simulink model "ChiefMaster_TTC580"  (R2022b)
settings: Solver=FixedStepAuto  StartTime=0.0  StopTime=10  FixedStep=0.01  RelTol=1e-3
values from neighbouring files (symbols this model uses):
  BattBox1_No = single(1)    [Parameters.m]
  BattBox2_No = single(2)    [Parameters.m]
  BattBox3_No = single(3)    [Parameters.m]
  CurrentLB = single(-3)    [Parameters.m]
  CurrentReductionConstant_Lvl0 = single(0.03)    [Parameters.m]
  CurrentReductionConstant_Lvl1 = single(0.05)    [Parameters.m]
  CurrentReductionConstant_Lvl2 = single(0.07)    [Parameters.m]
  CurrentReductionConstant_Lvl3 = single(0.1)    [Parameters.m]
  CurrentUB = single(3)    [Parameters.m]
  DCHV_Minus_In_Delay_ms = single(500)    [Parameters.m]
  FL_sHVC_CellBalanceVoltage_mV = single(3500)    [Parameters.m]
  FL_sInrushCurrent_dividebyzero = single(0.00001)    [Parameters.m]
  FL_u8HMI_BuzzerTimer = uint8(3)    [Parameters.m]
  IP_boActValue = true    [Parameters.m]
  IP_boDeactValue = false    [Parameters.m]
  IP_boInitValue = false    [Parameters.m]
  IP_s_LB = 18000    [Parameters.m]
  IP_s_UB = 22000    [Parameters.m]
  IP_sBatt1_ChargeCurrentMax_Factor = single(0.1)    [Parameters.m]
  IP_sBatt1_ChargeCurrentMax_LB = single(0)    [Parameters.m]
  IP_sBatt1_ChargeCurrentMax_Offset = single(0)    [Parameters.m]
  IP_sBatt1_ChargeCurrentMax_UB = single(6553.5)    [Parameters.m]
  IP_sBatt1_Current_Factor = single(0.1)    [Parameters.m]
  IP_sBatt1_Current_LB = single(-3276.8)    [Parameters.m]
  IP_sBatt1_Current_Offset = single(0)    [Parameters.m]
  IP_sBatt1_Current_UB = single(3276.8)    [Parameters.m]
  IP_sBatt1_DisChargeCurrentMax_Factor = single(0.1)    [Parameters.m]
  IP_sBatt1_DisChargeCurrentMax_LB = single(0)    [Parameters.m]
  IP_sBatt1_DisChargeCurrentMax_Offset = single(0)    [Parameters.m]
  IP_sBatt1_DisChargeCurrentMax_UB = single(6553.5)    [Parameters.m]
  IP_sBatt1_InsulationResistance_Factor = single(5)    [Parameters.m]
  IP_sBatt1_InsulationResistance_LB = single(0)    [Parameters.m]
  IP_sBatt1_InsulationResistance_Offset = single(0)    [Parameters.m]
  IP_sBatt1_InsulationResistance_UB = single(0)    [Parameters.m]
  IP_sBatt1_LiBa_IntResist_mOhm = single(25)    [Parameters.m]
  IP_sBatt1_SOC_Factor = single(1)    [Parameters.m]
  IP_sBatt1_SOC_LB = single(0)    [Parameters.m]
  IP_sBatt1_SOC_Offset = single(0)    [Parameters.m]
  IP_sBatt1_SOC_UB = single(100)    [Parameters.m]
  IP_sBatt1_SOH_Factor = single(1)    [Parameters.m]
  IP_sBatt1_SOH_LB = single(0)    [Parameters.m]
  IP_sBatt1_SOH_Offset = single(0)    [Parameters.m]
  IP_sBatt1_SOH_UB = single(100)    [Parameters.m]
  IP_sBatt1_Ubatt_Factor = single(0.1)    [Parameters.m]
  IP_sBatt1_Ubatt_LB = single(0)    [Parameters.m]
  IP_sBatt1_Ubatt_Offset = single(0)    [Parameters.m]
  IP_sBatt1_Ubatt_UB = single(6553.5)    [Parameters.m]
  IP_sBatt1_UserRi_Factor = single(1)    [Parameters.m]
  IP_sBatt1_UserRi_LB = single(0)    [Parameters.m]
  IP_sBatt1_UserRi_Offset = single(0)    [Parameters.m]
  IP_sBatt1_UserRi_UB = single(255)    [Parameters.m]
  IP_sBatt1_VoltageAtSensor_Factor = single(0.02)    [Parameters.m]
  IP_sBatt1_VoltageAtSensor_LB = single(0)    [Parameters.m]
  IP_sBatt1_VoltageAtSensor_Offset = single(0)    [Parameters.m]
  IP_sBatt1_VoltageAtSensor_UB = single(1310.7)    [Parameters.m]
  IP_sBatt2_LiBa_IntResist_mOhm = single(25)    [Parameters.m]
  IP_sBatt3_LiBa_IntResist_mOhm = single(25)    [Parameters.m]
  IP_sEM_LB = 2000    [Parameters.m]
  IP_sEM_UB = 8000    [Parameters.m]
  IP_sFB_LB = 5000    [Parameters.m]
  IP_sFB_UB = 10000    [Parameters.m]
  IP_sHVIL_LB = 12000    [Parameters.m]
  IP_sHVIL_UB = 15000    [Parameters.m]
  IP_sLoad_Voltage_Factor = single(1)    [Parameters.m]
  IP_sLoad_Voltage_LB = single(0)    [Parameters.m]
  IP_sLoad_Voltage_Offset = single(0)    [Parameters.m]
  IP_sLoad_Voltage_UB = single(65535)    [Parameters.m]
  IP_u8HVIL_Delay_ms = uint8(100)    [Parameters.m]
  IP_u8HW_IN_delay_ms = uint8(100)    [Parameters.m]
  IT_sInsulationSafeValue_kOhm = single(650)    [Parameters.m]
  IT_u8IMD_DelayTime_s = uint8(20)    [Parameters.m]
  MainHV_Minus_In_Delay = single(5)    [Parameters.m]
  MainHV_StatusDelay = single(5)    [Parameters.m]
  NotAvailable_uint16 = single(65535)    [Parameters.m]
  NotAvailable_uint8 = uint8(255)    [Parameters.m]
  OP_boHVIL_Supply = boolean(1)    [Parameters.m]
  SafeCurrentToCloseHV_A = single(5)    [Parameters.m]
  SafeVoltageToCloseHV_V = single(0.5)    [Parameters.m]
  UnexpectedBattChargingFcn_Available = boolean(1)    [Parameters.m]
  Voltage_NA_UB = uint16(65535)    [Parameters.m]
  VoltageSensorAvailableBB1 = boolean(0)    [Parameters.m]
  VoltageSensorAvailableBB2 = boolean(0)    [Parameters.m]
  VoltageSensorAvailableBB3 = boolean(0)    [Parameters.m]
libraries: simulink x184, Library_DataProcessing_v1_1 x167, Library_DataProcessing_v1 x142, libCM x28
(part 18 of 19)

== system ChiefMaster_TTC580/ChiefMaster/Input Processing/LiBa/LiBa_Box3/BMS_InsulationMonitor/Subsystem ==
  byte0 : Inport
  byte1 : Inport  Port=2
  C_LB_BMS_InsulationMonitor_Timeout : Inport  Port=3
  Bus Creator : BusCreator  Inputs=3
  Constant : Constant  OutDataTypeStr=single
  Constant1 : Constant  Value=0  OutDataTypeStr=single
  Constant2 : Constant  Value=0  OutDataTypeStr=single
  Constant3 : Constant  Value=65535  OutDataTypeStr=single
  Constant4 : Constant  Value=0  OutDataTypeStr=single
  Lib_2byte_ArthConcat : Library_DataProcessing_v1_1/Lib_2byte_ArthConcat  SystemSampleTime=-1  VariantActivationTime=update diagram  Latency=0  AutoFrameSizeCalculation=off
  Lib_InputProcessing+SafeValueSelector_Data : Library_DataProcessing_v1_1/Lib_InputProcessing+SafeValueSelector_Data  SystemSampleTime=-1  VariantActivationTime=update diagram  Latency=0  AutoFrameSizeCalculation=off
  IP_LB_BMS_Pack_Leak_Pos_Raw_mV_DataBus : Outport
  wires:
  Constant4/1 -> Lib_InputProcessing+SafeValueSelector_Data/7, Lib_InputProcessing+SafeValueSelector_Data/8
  Constant3/1 -> Lib_InputProcessing+SafeValueSelector_Data/6
  Constant2/1 -> Lib_InputProcessing+SafeValueSelector_Data/5
  Constant1/1 -> Lib_InputProcessing+SafeValueSelector_Data/4
  Constant/1 -> Lib_InputProcessing+SafeValueSelector_Data/3
  Bus Creator/1 -> IP_LB_BMS_Pack_Leak_Pos_Raw_mV_DataBus/1  "IP_LB_BMS_Pack_Leak_Pos_Raw_mV_DataBus"
  Lib_InputProcessing+SafeValueSelector_Data/3 -> Bus Creator/3
  Lib_InputProcessing+SafeValueSelector_Data/2 -> Bus Creator/2
  Lib_InputProcessing+SafeValueSelector_Data/1 -> Bus Creator/1
  C_LB_BMS_InsulationMonitor_Timeout/1 -> Lib_InputProcessing+SafeValueSelector_Data/2
  Lib_2byte_ArthConcat/1 -> Lib_InputProcessing+SafeValueSelector_Data/1
  byte1/1 -> Lib_2byte_ArthConcat/2
  byte0/1 -> Lib_2byte_ArthConcat/1

== system ChiefMaster_TTC580/ChiefMaster/Input Processing/LiBa/LiBa_Box3/BMS_InsulationMonitor/Subsystem1 ==
  byte2 : Inport
  byte3 : Inport  Port=2
  C_LB_BMS_InsulationMonitor_Timeout : Inport  Port=3
  Bus Creator : BusCreator  Inputs=3
  Constant : Constant  OutDataTypeStr=single
  Constant1 : Constant  Value=0  OutDataTypeStr=single
  Constant2 : Constant  Value=0  OutDataTypeStr=single
  Constant3 : Constant  Value=65535  OutDataTypeStr=single
  Constant4 : Constant  Value=0  OutDataTypeStr=single
  Lib_2byte_ArthConcat : Library_DataProcessing_v1_1/Lib_2byte_ArthConcat  SystemSampleTime=-1  VariantActivationTime=update diagram  Latency=0  AutoFrameSizeCalculation=off
  Lib_InputProcessing+SafeValueSelector_Data : Library_DataProcessing_v1_1/Lib_InputProcessing+SafeValueSelector_Data  SystemSampleTime=-1  VariantActivationTime=update diagram  Latency=0  AutoFrameSizeCalculation=off
  IP_LB_BMS_Pack_Leak_Neg_Raw_mV_DataBus : Outport
  wires:
  Bus Creator/1 -> IP_LB_BMS_Pack_Leak_Neg_Raw_mV_DataBus/1  "IP_LB_BMS_Pack_Leak_Neg_Raw_mV_DataBus"
  C_LB_BMS_InsulationMonitor_Timeout/1 -> Lib_InputProcessing+SafeValueSelector_Data/2
  byte3/1 -> Lib_2byte_ArthConcat/2
  byte2/1 -> Lib_2byte_ArthConcat/1
  Constant3/1 -> Lib_InputProcessing+SafeValueSelector_Data/6
  Constant2/1 -> Lib_InputProcessing+SafeValueSelector_Data/5
  Lib_InputProcessing+SafeValueSelector_Data/3 -> Bus Creator/3
  Lib_InputProcessing+SafeValueSelector_Data/2 -> Bus Creator/2
  Constant/1 -> Lib_InputProcessing+SafeValueSelector_Data/3
  Lib_InputProcessing+SafeValueSelector_Data/1 -> Bus Creator/1
  Constant1/1 -> Lib_InputProcessing+SafeValueSelector_Data/4
  Lib_2byte_ArthConcat/1 -> Lib_InputProcessing+SafeValueSelector_Data/1
  Constant4/1 -> Lib_InputProcessing+SafeValueSelector_Data/7, Lib_InputProcessing+SafeValueSelector_Data/8

== system ChiefMaster_TTC580/ChiefMaster/Input Processing/LiBa/LiBa_Box3/BMS_InsulationMonitor/Subsystem2 ==
  byte4 : Inport
  byte5 : Inport  Port=2
  C_LB_BMS_InsulationMonitor_Timeout : Inport  Port=3
  Bus Creator : BusCreator  Inputs=3
  Constant : Constant  OutDataTypeStr=single
  Constant1 : Constant  Value=0  OutDataTypeStr=single
  Constant2 : Constant  Value=0  OutDataTypeStr=single
  Constant3 : Constant  Value=65535  OutDataTypeStr=single
  Constant4 : Constant  Value=0  OutDataTypeStr=single
  Lib_2byte_ArthConcat : Library_DataProcessing_v1_1/Lib_2byte_ArthConcat  SystemSampleTime=-1  VariantActivationTime=update diagram  Latency=0  AutoFrameSizeCalculation=off
  Lib_InputProcessing+SafeValueSelector_Data : Library_DataProcessing_v1_1/Lib_InputProcessing+SafeValueSelector_Data  SystemSampleTime=-1  VariantActivationTime=update diagram  Latency=0  AutoFrameSizeCalculation=off
  IP_LB_BMS_Pack_Leak_Mid_Raw_mV_DataBus : Outport
  wires:
  byte5/1 -> Lib_2byte_ArthConcat/2
  byte4/1 -> Lib_2byte_ArthConcat/1
  C_LB_BMS_InsulationMonitor_Timeout/1 -> Lib_InputProcessing+SafeValueSelector_Data/2
  Bus Creator/1 -> IP_LB_BMS_Pack_Leak_Mid_Raw_mV_DataBus/1  "IP_LB_BMS_Pack_Leak_Mid_Raw_mV_DataBus"
  Lib_InputProcessing+SafeValueSelector_Data/1 -> Bus Creator/1
  Constant/1 -> Lib_InputProcessing+SafeValueSelector_Data/3
  Constant4/1 -> Lib_InputProcessing+SafeValueSelector_Data/7, Lib_InputProcessing+SafeValueSelector_Data/8
  Lib_InputProcessing+SafeValueSelector_Data/2 -> Bus Creator/2
  Constant1/1 -> Lib_InputProcessing+SafeValueSelector_Data/4
  Lib_2byte_ArthConcat/1 -> Lib_InputProcessing+SafeValueSelector_Data/1
  Lib_InputProcessing+SafeValueSelector_Data/3 -> Bus Creator/3
  Constant3/1 -> Lib_InputProcessing+SafeValueSelector_Data/6
  Constant2/1 -> Lib_InputProcessing+SafeValueSelector_Data/5

== system ChiefMaster_TTC580/ChiefMaster/Input Processing/LiBa/LiBa_Box3/BMS_Status01/Subsystem1 ==
  byte1 : Inport
  C_LB_BMS_Status01_Timeout : Inport  Port=2
  Bus Creator : BusCreator  Inputs=3
  Constant : Constant  OutDataTypeStr=single
  Constant1 : Constant  Value=0  OutDataTypeStr=single
  Constant2 : Constant  Value=0  OutDataTypeStr=single
  Constant3 : Constant  Value=255  OutDataTypeStr=single
  Constant4 : Constant  Value=0  OutDataTypeStr=single
  Lib_InputProcessing+SafeValueSelector_Data : Library_DataProcessing_v1_1/Lib_InputProcessing+SafeValueSelector_Data  SystemSampleTime=-1  VariantActivationTime=update diagram  Latency=0  AutoFrameSizeCalculation=off
  IP_LB_BMS_IO_state_Input_DataBus : Outport
  wires:
  byte1/1 -> Lib_InputProcessing+SafeValueSelector_Data/1
  Bus Creator/1 -> IP_LB_BMS_IO_state_Input_DataBus/1  "IP_LB_BMS_IO_state_Input_DataBus"
  C_LB_BMS_Status01_Timeout/1 -> Lib_InputProcessing+SafeValueSelector_Data/2
  Constant3/1 -> Lib_InputProcessing+SafeValueSelector_Data/6
  Constant2/1 -> Lib_InputProcessing+SafeValueSelector_Data/5
  Lib_InputProcessing+SafeValueSelector_Data/3 -> Bus Creator/3
  Lib_InputProcessing+SafeValueSelector_Data/2 -> Bus Creator/2
  Constant/1 -> Lib_InputProcessing+SafeValueSelector_Data/3
  Lib_InputProcessing+SafeValueSelector_Data/1 -> Bus Creator/1
  Constant1/1 -> Lib_InputProcessing+SafeValueSelector_Data/4
  Constant4/1 -> Lib_InputProcessing+SafeValueSelector_Data/7, Lib_InputProcessing+SafeValueSelector_Data/8

== system ChiefMaster_TTC580/ChiefMaster/Input Processing/LiBa/LiBa_Box3/BMS_Status01/Subsystem2 ==
  byte2 : Inport
  C_LB_BMS_Status01_Timeout : Inport  Port=2
  Bus Creator : BusCreator  Inputs=3
  Constant : Constant  OutDataTypeStr=single
  Constant1 : Constant  Value=0  OutDataTypeStr=single
  Constant2 : Constant  Value=0  OutDataTypeStr=single
  Constant3 : Constant  Value=255  OutDataTypeStr=single
  Constant4 : Constant  Value=0  OutDataTypeStr=single
  Lib_InputProcessing+SafeValueSelector_Data : Library_DataProcessing_v1_1/Lib_InputProcessing+SafeValueSelector_Data  SystemSampleTime=-1  VariantActivationTime=update diagram  Latency=0  AutoFrameSizeCalculation=off
  IP_LB_BMS_IO_State_Output_DataBus : Outport
  wires:
  byte2/1 -> Lib_InputProcessing+SafeValueSelector_Data/1
  C_LB_BMS_Status01_Timeout/1 -> Lib_InputProcessing+SafeValueSelector_Data/2
  Bus Creator/1 -> IP_LB_BMS_IO_State_Output_DataBus/1  "IP_LB_BMS_IO_State_Output_DataBus"
  Lib_InputProcessing+SafeValueSelector_Data/1 -> Bus Creator/1
  Constant/1 -> Lib_InputProcessing+SafeValueSelector_Data/3
  Constant4/1 -> Lib_InputProcessing+SafeValueSelector_Data/7, Lib_InputProcessing+SafeValueSelector_Data/8
  Lib_InputProcessing+SafeValueSelector_Data/2 -> Bus Creator/2
  Constant1/1 -> Lib_InputProcessing+SafeValueSelector_Data/4
  Lib_InputProcessing+SafeValueSelector_Data/3 -> Bus Creator/3
  Constant3/1 -> Lib_InputProcessing+SafeValueSelector_Data/6
  Constant2/1 -> Lib_InputProcessing+SafeValueSelector_Data/5

== system ChiefMaster_TTC580/ChiefMaster/Input Processing/LiBa/LiBa_Box3/BMS_Status01/Subsystem3 ==
  byte4 : Inport
  byte5 : Inport  Port=2
  C_LB_BMS_Status01_Timeout : Inport  Port=3
  Bus Creator : BusCreator  Inputs=3
  Constant : Constant  Value=0.1  OutDataTypeStr=single
  Constant1 : Constant  Value=0  OutDataTypeStr=single
  Constant2 : Constant  Value=0  OutDataTypeStr=single
  Constant3 : Constant  Value=6553.5  OutDataTypeStr=single
  Constant4 : Constant  Value=0  OutDataTypeStr=single
  Lib_2byte_ArthConcat : Library_DataProcessing_v1_1/Lib_2byte_ArthConcat  SystemSampleTime=-1  VariantActivationTime=update diagram  Latency=0  AutoFrameSizeCalculation=off
  Lib_InputProcessing+SafeValueSelector_Data : Library_DataProcessing_v1_1/Lib_InputProcessing+SafeValueSelector_Data  SystemSampleTime=-1  VariantActivationTime=update diagram  Latency=0  AutoFrameSizeCalculation=off
  IP_LB_BMS_DYN_Lim_Current_IN_A_DataBus : Outport
  wires:
  Bus Creator/1 -> IP_LB_BMS_DYN_Lim_Current_IN_A_DataBus/1  "IP_LB_BMS_DYN_Lim_Current_IN_A_DataBus"
  Constant3/1 -> Lib_InputProcessing+SafeValueSelector_Data/6
  Lib_2byte_ArthConcat/1 -> Lib_InputProcessing+SafeValueSelector_Data/1
  Constant1/1 -> Lib_InputProcessing+SafeValueSelector_Data/4
  Constant4/1 -> Lib_InputProcessing+SafeValueSelector_Data/8, Lib_InputProcessing+SafeValueSelector_Data/7
  Constant/1 -> Lib_InputProcessing+SafeValueSelector_Data/3
  Constant2/1 -> Lib_InputProcessing+SafeValueSelector_Data/5
  Lib_InputProcessing+SafeValueSelector_Data/1 -> Bus Creator/1
  Lib_InputProcessing+SafeValueSelector_Data/3 -> Bus Creator/3
  Lib_InputProcessing+SafeValueSelector_Data/2 -> Bus Creator/2
  byte4/1 -> Lib_2byte_ArthConcat/1
  byte5/1 -> Lib_2byte_ArthConcat/2
  C_LB_BMS_Status01_Timeout/1 -> Lib_InputProcessing+SafeValueSelector_Data/2

== system ChiefMaster_TTC580/ChiefMaster/Input Processing/LiBa/LiBa_Box3/BMS_Status01/Subsystem4 ==
  byte6 : Inport
  byte7 : Inport  Port=2
  C_LB_BMS_Status01_Timeout : Inport  Port=3
  Bus Creator : BusCreator  Inputs=3
  Constant : Constant  Value=0.1  OutDataTypeStr=single
  Constant1 : Constant  Value=0  OutDataTypeStr=single
  Constant2 : Constant  Value=0  OutDataTypeStr=single
  Constant3 : Constant  Value=6553.5  OutDataTypeStr=single
  Constant4 : Constant  Value=0  OutDataTypeStr=single
  Lib_2byte_ArthConcat : Library_DataProcessing_v1_1/Lib_2byte_ArthConcat  SystemSampleTime=-1  VariantActivationTime=update diagram  Latency=0  AutoFrameSizeCalculation=off
  Lib_InputProcessing+SafeValueSelector_Data : Library_DataProcessing_v1_1/Lib_InputProcessing+SafeValueSelector_Data  SystemSampleTime=-1  VariantActivationTime=update diagram  Latency=0  AutoFrameSizeCalculation=off
  IP_LB_BMS_DYN_Lim_Current_OUT_A_DataBus : Outport
  wires:
  C_LB_BMS_Status01_Timeout/1 -> Lib_InputProcessing+SafeValueSelector_Data/2
  byte7/1 -> Lib_2byte_ArthConcat/2
  byte6/1 -> Lib_2byte_ArthConcat/1
  Lib_InputProcessing+SafeValueSelector_Data/2 -> Bus Creator/2
  Lib_InputProcessing+SafeValueSelector_Data/3 -> Bus Creator/3
  Lib_InputProcessing+SafeValueSelector_Data/1 -> Bus Creator/1
  Constant2/1 -> Lib_InputProcessing+SafeValueSelector_Data/5
  Constant/1 -> Lib_InputProcessing+SafeValueSelector_Data/3
  Constant4/1 -> Lib_InputProcessing+SafeValueSelector_Data/7, Lib_InputProcessing+SafeValueSelector_Data/8
  Constant1/1 -> Lib_InputProcessing+SafeValueSelector_Data/4
  Lib_2byte_ArthConcat/1 -> Lib_InputProcessing+SafeValueSelector_Data/1
  Constant3/1 -> Lib_InputProcessing+SafeValueSelector_Data/6
  Bus Creator/1 -> IP_LB_BMS_DYN_Lim_Current_OUT_A_DataBus/1  "IP_LB_BMS_DYN_Lim_Current_OUT_A_DataBus"

== system ChiefMaster_TTC580/ChiefMaster/Input Processing/LiBa/LiBa_Box3/BMS_Status02/Subsystem1 ==
  byte2 : Inport
  byte3 : Inport  Port=2
  byte4 : Inport  Port=3
  byte5 : Inport  Port=4
  C_LB_BMS_Status02_Timeout : Inport  Port=5
  Bus Creator : BusCreator  Inputs=3
  Constant : Constant  Value=0.01  OutDataTypeStr=single
  Constant1 : Constant  Value=0  OutDataTypeStr=single
  Constant2 : Constant  Value=-21474836.48  OutDataTypeStr=single
  Constant3 : Constant  Value=21474836.47  OutDataTypeStr=single
  Constant4 : Constant  Value=0  OutDataTypeStr=single
  Data Type Conversion : DataTypeConversion  OutDataTypeStr=int32  SaturateOnIntegerOverflow=off  RndMeth=Floor
  Lib_4byte_ArthConcat : Library_DataProcessing_v1_1/Lib_4byte_ArthConcat  SystemSampleTime=-1  VariantActivationTime=update diagram  Latency=0  AutoFrameSizeCalculation=off
  Lib_InputProcessing+SafeValueSelector_Data : Library_DataProcessing_v1_1/Lib_InputProcessing+SafeValueSelector_Data  SystemSampleTime=-1  VariantActivationTime=update diagram  Latency=0  AutoFrameSizeCalculation=off
  IP_LB_BMS_Pack_Current_Master_mA_DataBus : Outport
  wires:
  Data Type Conversion/1 -> Lib_InputProcessing+SafeValueSelector_Data/1
  Bus Creator/1 -> IP_LB_BMS_Pack_Current_Master_mA_DataBus/1  "IP_LB_BMS_Pack_Current_Master_mA_DataBus"
  Constant3/1 -> Lib_InputProcessing+SafeValueSelector_Data/6
  Lib_4byte_ArthConcat/1 -> Data Type Conversion/1
  Constant1/1 -> Lib_InputProcessing+SafeValueSelector_Data/4
  Constant4/1 -> Lib_InputProcessing+SafeValueSelector_Data/8, Lib_InputProcessing+SafeValueSelector_Data/7
  Constant/1 -> Lib_InputProcessing+SafeValueSelector_Data/3
  Constant2/1 -> Lib_InputProcessing+SafeValueSelector_Data/5
  Lib_InputProcessing+SafeValueSelector_Data/1 -> Bus Creator/1
  Lib_InputProcessing+SafeValueSelector_Data/3 -> Bus Creator/3
  Lib_InputProcessing+SafeValueSelector_Data/2 -> Bus Creator/2
  byte2/1 -> Lib_4byte_ArthConcat/1
  byte3/1 -> Lib_4byte_ArthConcat/2
  C_LB_BMS_Status02_Timeout/1 -> Lib_InputProcessing+SafeValueSelector_Data/2
  byte4/1 -> Lib_4byte_ArthConcat/3
  byte5/1 -> Lib_4byte_ArthConcat/4

== system ChiefMaster_TTC580/ChiefMaster/Input Processing/LiBa/LiBa_Box3/BMS_Status02/Subsystem2 ==
  byte6 : Inport
  byte7 : Inport  Port=2
  C_LB_BMS_Status02_Timeout : Inport  Port=3
  Bus Creator : BusCreator  Inputs=3
  Constant : Constant  Value=0.1  OutDataTypeStr=single
  Constant1 : Constant  Value=0  OutDataTypeStr=single
  Constant2 : Constant  Value=0  OutDataTypeStr=single
  Constant3 : Constant  Value=6553.5  OutDataTypeStr=single
  Constant4 : Constant  Value=0  OutDataTypeStr=single
  Lib_2byte_ArthConcat : Library_DataProcessing_v1_1/Lib_2byte_ArthConcat  SystemSampleTime=-1  VariantActivationTime=update diagram  Latency=0  AutoFrameSizeCalculation=off
  Lib_InputProcessing+SafeValueSelector_Data : Library_DataProcessing_v1_1/Lib_InputProcessing+SafeValueSelector_Data  SystemSampleTime=-1  VariantActivationTime=update diagram  Latency=0  AutoFrameSizeCalculation=off
  IP_LB_BMS_Pack_V_Cells_DataBus : Outport
  wires:
  Lib_2byte_ArthConcat/1 -> Lib_InputProcessing+SafeValueSelector_Data/1
  Bus Creator/1 -> IP_LB_BMS_Pack_V_Cells_DataBus/1  "IP_LB_BMS_Pack_V_Cells_DataBus"
  Constant3/1 -> Lib_InputProcessing+SafeValueSelector_Data/6
  Constant1/1 -> Lib_InputProcessing+SafeValueSelector_Data/4
  Constant4/1 -> Lib_InputProcessing+SafeValueSelector_Data/8, Lib_InputProcessing+SafeValueSelector_Data/7
  Constant/1 -> Lib_InputProcessing+SafeValueSelector_Data/3
  Constant2/1 -> Lib_InputProcessing+SafeValueSelector_Data/5
  Lib_InputProcessing+SafeValueSelector_Data/1 -> Bus Creator/1
  Lib_InputProcessing+SafeValueSelector_Data/3 -> Bus Creator/3
  Lib_InputProcessing+SafeValueSelector_Data/2 -> Bus Creator/2
  byte6/1 -> Lib_2byte_ArthConcat/1
  byte7/1 -> Lib_2byte_ArthConcat/2
  C_LB_BMS_Status02_Timeout/1 -> Lib_InputProcessing+SafeValueSelector_Data/2

== system ChiefMaster_TTC580/ChiefMaster/Input Processing/LiBa/LiBa_Box3/BMS_Status02/Subsystem3 ==
  byte0 : Inport
  byte1 : Inport  Port=2
  C_LB_BMS_Status02_Timeout : Inport  Port=3
  Bus Creator : BusCreator  Inputs=3
  Constant : Constant  Value=0.01  OutDataTypeStr=single
  Constant1 : Constant  Value=0  OutDataTypeStr=single
  Constant2 : Constant  Value=-327.68  OutDataTypeStr=single
  Constant3 : Constant  Value=327.67  OutDataTypeStr=single
  Constant4 : Constant  Value=0  OutDataTypeStr=single
  Data Type Conversion : DataTypeConversion  OutDataTypeStr=int16  SaturateOnIntegerOverflow=off  RndMeth=Floor
  Lib_2byte_ArthConcat : Library_DataProcessing_v1_1/Lib_2byte_ArthConcat  SystemSampleTime=-1  VariantActivationTime=update diagram  Latency=0  AutoFrameSizeCalculation=off
  Lib_InputProcessing+SafeValueSelector_Data : Library_DataProcessing_v1_1/Lib_InputProcessing+SafeValueSelector_Data  SystemSampleTime=-1  VariantActivationTime=update diagram  Latency=0  AutoFrameSizeCalculation=off
  IP_LB_BMS_Pack_Q_SOC_Internal_DataBus : Outport
  wires:
  C_LB_BMS_Status02_Timeout/1 -> Lib_InputProcessing+SafeValueSelector_Data/2
  byte1/1 -> Lib_2byte_ArthConcat/2
  byte0/1 -> Lib_2byte_ArthConcat/1
  Lib_InputProcessing+SafeValueSelector_Data/2 -> Bus Creator/2
  Lib_InputProcessing+SafeValueSelector_Data/3 -> Bus Creator/3
  Lib_InputProcessing+SafeValueSelector_Data/1 -> Bus Creator/1
  Constant2/1 -> Lib_InputProcessing+SafeValueSelector_Data/5
  Constant/1 -> Lib_InputProcessing+SafeValueSelector_Data/3
  Constant4/1 -> Lib_InputProcessing+SafeValueSelector_Data/7, Lib_InputProcessing+SafeValueSelector_Data/8
  Constant1/1 -> Lib_InputProcessing+SafeValueSelector_Data/4
  Lib_2byte_ArthConcat/1 -> Data Type Conversion/1
  Constant3/1 -> Lib_InputProcessing+SafeValueSelector_Data/6
  Bus Creator/1 -> IP_LB_BMS_Pack_Q_SOC_Internal_DataBus/1  "IP_LB_BMS_Pack_Q_SOC_Internal_DataBus"
  Data Type Conversion/1 -> Lib_InputProcessing+SafeValueSelector_Data/1

== system ChiefMaster_TTC580/ChiefMaster/Input Processing/LiBa/LiBa_Box3/BMS_Status03/Subsystem3 ==
  byte0 : Inport
  byte1 : Inport  Port=2
  C_LB_BMS_Status03_Timeout : Inport  Port=3
  Bus Creator : BusCreator  Inputs=3
  Constant : Constant  Value=0.1  OutDataTypeStr=single
  Constant1 : Constant  Value=0  OutDataTypeStr=single
  Constant2 : Constant  Value=0  OutDataTypeStr=single
  Constant3 : Constant  Value=6553.5  OutDataTypeStr=single
  Constant4 : Constant  Value=0  OutDataTypeStr=single
  Lib_2byte_ArthConcat : Library_DataProcessing_v1_1/Lib_2byte_ArthConcat  SystemSampleTime=-1  VariantActivationTime=update diagram  Latency=0  AutoFrameSizeCalculation=off
  Lib_InputProcessing+SafeValueSelector_Data : Library_DataProcessing_v1_1/Lib_InputProcessing+SafeValueSelector_Data  SystemSampleTime=-1  VariantActivationTime=update diagram  Latency=0  AutoFrameSizeCalculation=off
  IP_LB_BMS_REQ_Charger_Current_A_DataBus : Outport
  wires:
  Lib_2byte_ArthConcat/1 -> Lib_InputProcessing+SafeValueSelector_Data/1
  Bus Creator/1 -> IP_LB_BMS_REQ_Charger_Current_A_DataBus/1  "IP_LB_BMS_REQ_Charger_Current_A_DataBus"
  Constant3/1 -> Lib_InputProcessing+SafeValueSelector_Data/6
  Constant1/1 -> Lib_InputProcessing+SafeValueSelector_Data/4
  Constant4/1 -> Lib_InputProcessing+SafeValueSelector_Data/8, Lib_InputProcessing+SafeValueSelector_Data/7
  Constant/1 -> Lib_InputProcessing+SafeValueSelector_Data/3
  Constant2/1 -> Lib_InputProcessing+SafeValueSelector_Data/5
  Lib_InputProcessing+SafeValueSelector_Data/1 -> Bus Creator/1
  Lib_InputProcessing+SafeValueSelector_Data/3 -> Bus Creator/3
  Lib_InputProcessing+SafeValueSelector_Data/2 -> Bus Creator/2
  byte0/1 -> Lib_2byte_ArthConcat/1
  byte1/1 -> Lib_2byte_ArthConcat/2
  C_LB_BMS_Status03_Timeout/1 -> Lib_InputProcessing+SafeValueSelector_Data/2

== system ChiefMaster_TTC580/ChiefMaster/Input Translation/Battery Signals/Subsystem12/Subsystem1/Subsystem1 ==
  <IP_LB_BMS_Pack_Leak_Pos_Raw_mV_DataBus> : Inport
  <IP_LB_BMS_Pack_Leak_Neg_Raw_mV_DataBus> : Inport  Port=2
  <IP_LB_BMS_Pack_V_Cells_DataBus> : Inport  Port=3
  AND : Logic  AllPortsSameDT=off  OutDataTypeStr=boolean
  Abs : Abs  SaturateOnIntegerOverflow=off
  Abs1 : Abs  SaturateOnIntegerOverflow=off
  Bus Selector{,1..3} (4 alike) : BusSelector  OutputSignals=sData
  Constant1 : Constant  Value=10  OutDataTypeStr=single
  Constant2 : Constant  Value=2000  OutDataTypeStr=single
  Constant3 : Constant  Value=IT_sInsulationSafeValue_kOhm  OutDataTypeStr=single
  Constant4 : Constant  Value=2.480  OutDataTypeStr=single
  Constant5 : Constant  Value=2.480  OutDataTypeStr=single
  Constant6 : Constant  Value=10  OutDataTypeStr=single
  Constant7 : Constant  Value=2000  OutDataTypeStr=single
  Constant8 : Constant  Value=IT_sInsulationSafeValue_kOhm  OutDataTypeStr=single
  Divide : Product  Inputs=*/
  Divide1 : Product  Inputs=*/
  GreaterThan : RelationalOperator  OutDataTypeStr=boolean  RndMeth=Simplest  InputSameDT=off
  GreaterThan1 : RelationalOperator  OutDataTypeStr=boolean  RndMeth=Simplest  InputSameDT=off
  Product : Product
  Product1 : Product
  Subtract{,1..3} (4 alike) : Sum  Inputs=+-
  mV to V : Gain  Gain=1/1000
  mV to V1 : Gain  Gain=1/1000
  IP_sLiBa_InsulationRes_Plus_kOhm : Outport
  IP_sLiBa_InsulationRes_Minus_kOhm : Outport  Port=2
  IP_LiBa_Insulation_Ok_Batt : Outport  Port=3
  wires:
  Constant5/1 -> Subtract2/2
  Constant2/1 -> Subtract1/2
  <IP_LB_BMS_Pack_Leak_Pos_Raw_mV_DataBus>/1 -> Bus Selector1/1
  Divide1/1 -> Subtract3/1
  Constant1/1 -> Product/2
  GreaterThan/1 -> AND/1
  mV to V1/1 -> Subtract2/1
  Divide/1 -> Subtract1/1
  Subtract3/1 -> IP_sLiBa_InsulationRes_Minus_kOhm/1, GreaterThan1/1
  Product1/1 -> Divide1/1
  GreaterThan1/1 -> AND/2
  Bus Selector2/1 -> Product1/1  "<sData>"
  Bus Selector1/1 -> mV to V/1  "<sData>"
  Subtract2/1 -> Abs1/1
  Bus Selector/1 -> Product/1  "<sData>"
  <IP_LB_BMS_Pack_Leak_Neg_Raw_mV_DataBus>/1 -> Bus Selector3/1
  Constant6/1 -> Product1/2
  <IP_LB_BMS_Pack_V_Cells_DataBus>/1 -> Bus Selector2/1, Bus Selector/1
  Constant7/1 -> Subtract3/2
  Constant8/1 -> GreaterThan1/2
  Constant3/1 -> GreaterThan/2
  Subtract1/1 -> IP_sLiBa_InsulationRes_Plus_kOhm/1, GreaterThan/1
  Bus Selector3/1 -> mV to V1/1  "<sData>"
  Abs1/1 -> Divide1/2
  Constant4/1 -> Subtract/2
  Product/1 -> Divide/1
  Abs/1 -> Divide/2
  Subtract/1 -> Abs/1
  mV to V/1 -> Subtract/1
  AND/1 -> IP_LiBa_Insulation_Ok_Batt/1  "IP_LiBa_Insulation_Ok_Batt"

== system ChiefMaster_TTC580/ChiefMaster/Input Translation/Battery Signals/Subsystem12/Subsystem2/Subsystem1 ==
  <IP_LB_BMS_Pack_Leak_Pos_Raw_mV_DataBus> : Inport
  <IP_LB_BMS_Pack_Leak_Neg_Raw_mV_DataBus> : Inport  Port=2
  <IP_LB_BMS_Pack_V_Cells_DataBus> : Inport  Port=3
  AND : Logic  AllPortsSameDT=off  OutDataTypeStr=boolean
  Abs : Abs  SaturateOnIntegerOverflow=off
  Abs1 : Abs  SaturateOnIntegerOverflow=off
  Bus Selector{,1..3} (4 alike) : BusSelector  OutputSignals=sData
  Constant1 : Constant  Value=10  OutDataTypeStr=single
  Constant2 : Constant  Value=2000  OutDataTypeStr=single
  Constant3 : Constant  Value=IT_sInsulationSafeValue_kOhm  OutDataTypeStr=single
  Constant4 : Constant  Value=2.480  OutDataTypeStr=single
  Constant5 : Constant  Value=2.480  OutDataTypeStr=single
  Constant6 : Constant  Value=10  OutDataTypeStr=single
  Constant7 : Constant  Value=2000  OutDataTypeStr=single
  Constant8 : Constant  Value=IT_sInsulationSafeValue_kOhm  OutDataTypeStr=single
  Divide : Product  Inputs=*/
  Divide1 : Product  Inputs=*/
  GreaterThan : RelationalOperator  OutDataTypeStr=boolean  RndMeth=Simplest  InputSameDT=off
  GreaterThan1 : RelationalOperator  OutDataTypeStr=boolean  RndMeth=Simplest  InputSameDT=off
  Product : Product
  Product1 : Product
  Subtract{,1..3} (4 alike) : Sum  Inputs=+-
  mV to V : Gain  Gain=1/1000
  mV to V1 : Gain  Gain=1/1000
  IP_sLiBa_InsulationRes_Plus_kOhm : Outport
  IP_sLiBa_InsulationRes_Minus_kOhm : Outport  Port=2
  IP_LiBa_Insulation_Ok_Batt : Outport  Port=3
  wires:
  Constant5/1 -> Subtract2/2
  Constant2/1 -> Subtract1/2
  <IP_LB_BMS_Pack_Leak_Pos_Raw_mV_DataBus>/1 -> Bus Selector1/1
  Divide1/1 -> Subtract3/1
  Constant1/1 -> Product/2
  GreaterThan/1 -> AND/1
  mV to V1/1 -> Subtract2/1
  Divide/1 -> Subtract1/1
  Subtract3/1 -> IP_sLiBa_InsulationRes_Minus_kOhm/1, GreaterThan1/1
  Product1/1 -> Divide1/1
  GreaterThan1/1 -> AND/2
  Bus Selector2/1 -> Product1/1  "<sData>"
  Bus Selector1/1 -> mV to V/1  "<sData>"
  Subtract2/1 -> Abs1/1
  Bus Selector/1 -> Product/1  "<sData>"
  <IP_LB_BMS_Pack_Leak_Neg_Raw_mV_DataBus>/1 -> Bus Selector3/1
  Constant6/1 -> Product1/2
  <IP_LB_BMS_Pack_V_Cells_DataBus>/1 -> Bus Selector2/1, Bus Selector/1
  Constant7/1 -> Subtract3/2
  Constant8/1 -> GreaterThan1/2
  Constant3/1 -> GreaterThan/2
  Subtract1/1 -> IP_sLiBa_InsulationRes_Plus_kOhm/1, GreaterThan/1
  Bus Selector3/1 -> mV to V1/1  "<sData>"
  Abs1/1 -> Divide1/2
  Constant4/1 -> Subtract/2
  Product/1 -> Divide/1
  Abs/1 -> Divide/2
  Subtract/1 -> Abs/1
  mV to V/1 -> Subtract/1
  AND/1 -> IP_LiBa_Insulation_Ok_Batt/1  "IP_LiBa_Insulation_Ok_Batt"

== system ChiefMaster_TTC580/ChiefMaster/Input Translation/Battery Signals/Subsystem12/Subsystem3/Subsystem1 ==
  <IP_LB_BMS_Pack_Leak_Pos_Raw_mV_DataBus> : Inport
  <IP_LB_BMS_Pack_Leak_Neg_Raw_mV_DataBus> : Inport  Port=2
  <IP_LB_BMS_Pack_V_Cells_DataBus> : Inport  Port=3
  AND : Logic  AllPortsSameDT=off  OutDataTypeStr=boolean
  Abs : Abs  SaturateOnIntegerOverflow=off
  Abs1 : Abs  SaturateOnIntegerOverflow=off
  Bus Selector{,1..3} (4 alike) : BusSelector  OutputSignals=sData
  Constant1 : Constant  Value=10  OutDataTypeStr=single
  Constant2 : Constant  Value=2000  OutDataTypeStr=single
  Constant3 : Constant  Value=IT_sInsulationSafeValue_kOhm  OutDataTypeStr=single
  Constant4 : Constant  Value=2.480  OutDataTypeStr=single
  Constant5 : Constant  Value=2.480  OutDataTypeStr=single
  Constant6 : Constant  Value=10  OutDataTypeStr=single
  Constant7 : Constant  Value=2000  OutDataTypeStr=single
  Constant8 : Constant  Value=IT_sInsulationSafeValue_kOhm  OutDataTypeStr=single
  Divide : Product  Inputs=*/
  Divide1 : Product  Inputs=*/
  GreaterThan : RelationalOperator  OutDataTypeStr=boolean  RndMeth=Simplest  InputSameDT=off
  GreaterThan1 : RelationalOperator  OutDataTypeStr=boolean  RndMeth=Simplest  InputSameDT=off
  Product : Product
  Product1 : Product
  Subtract{,1..3} (4 alike) : Sum  Inputs=+-
  mV to V : Gain  Gain=1/1000
  mV to V1 : Gain  Gain=1/1000
  IP_sLiBa_InsulationRes_Plus_kOhm : Outport
  IP_sLiBa_InsulationRes_Minus_kOhm : Outport  Port=2
  IP_LiBa_Insulation_Ok_Batt : Outport  Port=3
  wires:
  Constant5/1 -> Subtract2/2
  Constant2/1 -> Subtract1/2
  <IP_LB_BMS_Pack_Leak_Pos_Raw_mV_DataBus>/1 -> Bus Selector1/1
  Divide1/1 -> Subtract3/1
  Constant1/1 -> Product/2
  GreaterThan/1 -> AND/1
  mV to V1/1 -> Subtract2/1
  Divide/1 -> Subtract1/1
  Subtract3/1 -> IP_sLiBa_InsulationRes_Minus_kOhm/1, GreaterThan1/1
  Product1/1 -> Divide1/1
  GreaterThan1/1 -> AND/2
  Bus Selector2/1 -> Product1/1  "<sData>"
  Bus Selector1/1 -> mV to V/1  "<sData>"
  Subtract2/1 -> Abs1/1
  Bus Selector/1 -> Product/1  "<sData>"
  <IP_LB_BMS_Pack_Leak_Neg_Raw_mV_DataBus>/1 -> Bus Selector3/1
  Constant6/1 -> Product1/2
  <IP_LB_BMS_Pack_V_Cells_DataBus>/1 -> Bus Selector2/1, Bus Selector/1
  Constant7/1 -> Subtract3/2
  Constant8/1 -> GreaterThan1/2
  Constant3/1 -> GreaterThan/2
  Subtract1/1 -> IP_sLiBa_InsulationRes_Plus_kOhm/1, GreaterThan/1
  Bus Selector3/1 -> mV to V1/1  "<sData>"
  Abs1/1 -> Divide1/2
  Constant4/1 -> Subtract/2
  Product/1 -> Divide/1
  Abs/1 -> Divide/2
  Subtract/1 -> Abs/1
  mV to V/1 -> Subtract/1
  AND/1 -> IP_LiBa_Insulation_Ok_Batt/1  "IP_LiBa_Insulation_OK_Batt"

== system ChiefMaster_TTC580/ChiefMaster/Output Processing/CM_OBD/CM_SystemStatus1_Msg3/Subsystem/Subsystem12 ==
  FL_sHVC_CellBalanceVoltage_mV : Inport
  IP_DataBus : Inport  Port=2
  Bus Selector4 : BusSelector  OutputSignals=FL_Databus.IT_Databus.IT_BatterySignal_Databus.IP_sBMS_MinCellVoltage_BB1,FL_Databus.IT_Databus.IT_BatterySignal_Databus.IT_boBMS_HV_REL_ON_BB1,FL_Databus.IT_Databus.IT_BatterySignal_Databus.IP_sBMS_MinCellVoltage_BB2,FL_Databus.IT_Databus.IT_BatterySignal_Databus.IT_boBMS_HV_REL_ON_BB2,FL_Databus.IT_Databus.IT_BatterySignal_Databus.IP_sBMS_MinCellVoltage_BB3,FL_Databus.IT_Databus.IT_BatterySignal_Databus.IT_boBMS_HV_REL_ON_BB3
  Switch : Switch  Criteria=u2 > Threshold  SaturateOnIntegerOverflow=off  InputSameDT=off
  Switch1 : Switch  Criteria=u2 > Threshold  SaturateOnIntegerOverflow=off  InputSameDT=off
  Switch2 : Switch  Criteria=u2 > Threshold  SaturateOnIntegerOverflow=off  InputSameDT=off
  Batt1_UCellMin : Outport
  Batt2_UCellMin : Outport  Port=2
  Batt3_UCellMin : Outport  Port=3
  wires:
  Switch2/1 -> Batt3_UCellMin/1
  Switch1/1 -> Batt2_UCellMin/1
  Switch/1 -> Batt1_UCellMin/1
  FL_sHVC_CellBalanceVoltage_mV/1 -> Switch2/3, Switch1/3, Switch/3
  Bus Selector4/5 -> Switch2/1  "<IP_sBMS_MinCellVoltage_BB3>"
  Bus Selector4/6 -> Switch2/2  "<IT_boBMS_HV_REL_ON_BB3>"
  Bus Selector4/3 -> Switch1/1  "<IP_sBMS_MinCellVoltage_BB2>"
  Bus Selector4/4 -> Switch1/2  "<IT_boBMS_HV_REL_ON_BB2>"
  Bus Selector4/1 -> Switch/1  "<IP_sBMS_MinCellVoltage_BB1>"
  Bus Selector4/2 -> Switch/2  "<IT_boBMS_HV_REL_ON_BB1>"
  IP_DataBus/1 -> Bus Selector4/1

== stateflow chart ChiefMaster_TTC580/ChiefMaster/Input Processing/HW Inputs/Subsystem/Input_Delay ==
  state Initial
    out = true;
  state After_delay
    out = Input;
  (default) -> Initial
  Initial -> After_delay : [after(IP_u8HW_IN_delay_ms, msec)]
  data: out output; IP_u8HW_IN_delay_ms input; Input input

== stateflow chart ChiefMaster_TTC580/ChiefMaster/Flow Logic/BDU Control/BDUSystem/delay ==
  state Default
    Out = false
  state hold
    Out = false
  state Actual
    Out = In
  (default) -> Default
  (junction 15) -> Default : [In == false]
  Default -> hold : [In == true]
  hold -> (junction 15) [order 2]
  Actual -> (junction 15)
  hold -> Actual [order 1] : after(DelayTime_s,sec)
  data: In input boolean; Out output boolean; DelayTime_s input

== stateflow chart ChiefMaster_TTC580/ChiefMaster/Input Translation/Battery Selection/ChartBatt1 ==
  state Default
    BattSelect=0;
  state Actia
    BattSelect=1;
  state LiBa
    BattSelect = 2;
  (default) -> Default
  Default -> Actia [order 1] : [BattAvailable_Actia == true &&...
      | BattAvailable_LiBa == false]
  Actia -> Default : [BattAvailable_Actia == false]
  Default -> LiBa [order 2] : [BattAvailable_Actia == false &&...
      | BattAvailable_LiBa == true]
  LiBa -> Default : [BattAvailable_LiBa == false]
  data: BattAvailable_LiBa input; BattAvailable_Actia input; BattSelect output

== stateflow chart ChiefMaster_TTC580/ChiefMaster/Flow Logic/BDU Control/BDUSystem/Chart_REQ_MAIN_Precharge ==
  state Default
    REQ_MainHV_ON_Precharge = false
  state PrechargeEnable
    REQ_MainHV_ON_Precharge = true
  state PrechargeDisable
    REQ_MainHV_ON_Precharge = false
  (default) -> Default
  Default -> PrechargeEnable : [MainHV_Minus_Status == 2 &&...
      | KL15_CM_disable == false]
  PrechargeDisable -> Default : [KL15_CM_disable == true ||...
      | (MainHV_Minus_Status == 1 || MainHV_Minus_Status == 3)]
  PrechargeEnable -> PrechargeDisable : [System_SD == true ||...
      | (MainHV_Plus_Status == 2 || MainHV_Plus_Status == 3) ||...
      | (MainHV_Minus_Status == 1 || MainHV_Minus_Status == 3)]
  data: REQ_MainHV_ON_Precharge output; MainHV_Minus_Status input; KL15_CM_disable input; System_SD input boolean; MainHV_Plus_Status input

== stateflow chart ChiefMaster_TTC580/ChiefMaster/Flow Logic/BDU Control/BDUSystem/Chart_REQ_MAIN_MINUS ==
  state Default
    REQ_MainHV_ON_MINUS = false
  state Hold
  state RELMinusClose
    REQ_MainHV_ON_MINUS = true
  (default) -> Default
  Default -> RELMinusClose : [after(5,sec) &&...
      | System_ESD == false &&...
      | System_SD == false &&...
      | KL15_CM_disable == false &&...
      | Reset == false &&...
      | In == true]
  (junction 36) -> Default : [System_ESD == true]
  Hold -> Default [order 1] : [CM_SafeToSD == true]
  Hold -> (junction 36) [order 2] : [after(5,sec)]
  RELMinusClose -> Hold : [System_SD == true ||...
      | KL15_CM_disable == true ||...
      | Reset == true]
  data: REQ_MainHV_ON_MINUS output; In input; CM_SafeToSD input; KL15_CM_disable input; System_ESD input; System_SD input; Reset input

== stateflow chart ChiefMaster_TTC580/ChiefMaster/Flow Logic/BDU Control/BDUSystem/Chart_PrechargeStatus ==
  state Default
    Precharge_Satus = 0
  state delay1
  state PrechargeSuccess
    Precharge_Satus = 1
  state PrechargeFail
    Precharge_Satus = 2
  (default) -> Default
  (junction 44) -> Default : [MainHV_Minus_Status == 1 ||...
      | MainHV_Minus_Status == 3]
  Default -> delay1 : [REQ_MainHV_ON_Precharge == true &&...
      | KL15_CM_diable == false]
  (junction 33) -> Default : [KL15_CM_diable == true]
  delay1 -> PrechargeFail [order 2] : [after(3,sec)]
  delay1 -> PrechargeSuccess [order 1] : [after(500,msec) &&...
      | LoadCurrent == 0 &&...
      | abs(LoadVoltage - SystemVoltage) <= 5]
  PrechargeFail -> (junction 36)
  PrechargeSuccess -> (junction 31)
  (junction 31) -> (junction 44)
  (junction 36) -> (junction 33)
  data: REQ_MainHV_ON_Precharge input; LoadCurrent input; LoadVoltage input; SystemVoltage input; KL15_CM_diable input; MainHV_Minus_Status input; Precharge_Satus output

== stateflow chart ChiefMaster_TTC580/ChiefMaster/Input Translation/Battery Selection/Chartbatt2 ==
  state Default
    BattSelect=0;
  state Actia
    BattSelect=1;
  state LiBa
    BattSelect = 2;
  (default) -> Default
  Default -> Actia [order 1] : [BattAvailable_Actia == true &&...
      | BattAvailable_LiBa == false]
  Actia -> Default : [BattAvailable_Actia == false]
  Default -> LiBa [order 2] : [BattAvailable_Actia == false &&...
      | BattAvailable_LiBa == true]
  LiBa -> Default : [BattAvailable_LiBa == false]
  data: BattAvailable_LiBa input; BattAvailable_Actia input; BattSelect output

== stateflow chart ChiefMaster_TTC580/ChiefMaster/Input Translation/Battery Selection/ChartBatt3 ==
  state Default
    BattSelect=0;
  state Actia
    BattSelect=1;
  state LiBa
    BattSelect = 2;
  (default) -> Default
  Default -> Actia [order 1] : [BattAvailable_Actia == true &&...
      | BattAvailable_LiBa == false]
  Actia -> Default : [BattAvailable_Actia == false]
  Default -> LiBa [order 2] : [BattAvailable_Actia == false &&...
      | BattAvailable_LiBa == true]
  LiBa -> Default : [BattAvailable_LiBa == false]
  data: BattAvailable_LiBa input; BattAvailable_Actia input; BattSelect output

== stateflow chart ChiefMaster_TTC580/ChiefMaster/Flow Logic/System Status/SDError/IMD_SD/Chart ==
  state Default
    IMD_Error=false;
  state IsoMonitorCheck
    IMD_Error=false;
  state IsoMonitorError
    IMD_Error=true;
  (default) -> Default
  Default -> IsoMonitorCheck : [IP_boBMS_InsulationReadyOK == true]
  IsoMonitorCheck -> IsoMonitorError : [IP_boBMS_InsulationSDError == true]
  data: IP_boBMS_InsulationReadyOK input; IP_boBMS_InsulationSDError input; IMD_Error output

== stateflow chart ChiefMaster_TTC580/ChiefMaster/Flow Logic/System Status/SDError/IMD_SD/Chart1 ==
  state Default
    IMD_Error=false;
  state IsoMonitorCheck
    IMD_Error=false;
  state IsoMonitorError
    IMD_Error=true;
  (default) -> Default
  Default -> IsoMonitorCheck : [IP_boBMS_InsulationReadyOK == true]
  IsoMonitorCheck -> IsoMonitorError : [IP_boBMS_InsulationSDError == true]
  data: IP_boBMS_InsulationReadyOK input; IP_boBMS_InsulationSDError input; IMD_Error output

== stateflow chart ChiefMaster_TTC580/ChiefMaster/Flow Logic/System Status/SDError/IMD_SD/Chart2 ==
  state Default
    IMD_Error=false;
  state IsoMonitorCheck
    IMD_Error=false;
  state IsoMonitorError
    IMD_Error=true;
  (default) -> Default
  Default -> IsoMonitorCheck : [IP_boBMS_InsulationReadyOK == true]
  IsoMonitorCheck -> IsoMonitorError : [IP_boBMS_InsulationSDError == true]
  data: IP_boBMS_InsulationReadyOK input; IP_boBMS_InsulationSDError input; IMD_Error output

== stateflow chart ChiefMaster_TTC580/ChiefMaster/Flow Logic/System Status/CMState/CMState ==
  state Sleep
    CMState=0;
  state ON
    state KL15ON
      CMState=1;
    state ISOMonitor_check
      CMState=2;
    state ISOMonitor_OK
      CMState=3;
    state BattRelayClose_Req
      CMState=4;
    state BattRelayClose
      CMState=5;
    state BDURelayClose_Req
      CMState=6;
    state BDURelayClose
      CMState=7;
    (default) -> KL15ON
    KL15ON -> ISOMonitor_check : [KL15_AllBoxes==true && IMD_Available == true]
    ISOMonitor_check -> ISOMonitor_OK : [InsulationReadyOK==true]
    ISOMonitor_OK -> BattRelayClose_Req : [BattRelay_Close_Req==true]
    BattRelayClose -> BattRelayClose_Req [order 2] : [BattRelay_Closed==false]
    BattRelayClose_Req -> BattRelayClose : [BattRelay_Closed==true]
    BattRelayClose -> BDURelayClose_Req [order 1] : [FL_boREQ_MainHV_ON_MINUS == true]
    BDURelayClose_Req -> BDURelayClose : [MainHV_Plus_Status == 2]
  state OFF
    state BDURelayOpen_Req
      CMState=8;
    state BDURelayOpen
      CMState=9;
    state BattRelayOpen_Req
      CMState=10;
    state BattRelayOpen
      CMState=11;
    state ISOMonitorOFF
      CMState=12;
    state KL15OFF
      CMState=13;
    (default) -> BDURelayOpen_Req
    BDURelayOpen_Req -> BDURelayOpen : [MainHV_Plus_Status==0]
    BDURelayOpen -> BattRelayOpen_Req : [BattRelay_Close_Req==false]
    BattRelayOpen_Req -> BattRelayOpen : [BattRelay_Closed==false]
    BattRelayOpen -> ISOMonitorOFF : [REQ_IMD_ON == false]
    ISOMonitorOFF -> KL15OFF : [KL15_AllBoxes==false]
  state Error
    CMState=14;
  (default) -> Sleep
  Sleep -> ON : [KL15==true]
  OFF -> Sleep [order 1] : [CMState==13]
  ON -> OFF [order 1] : [KL15==false]
  Error -> ON [order 1] : [ShutdownError == false &&...
      | KL15==true]
  ON -> Error [order 2] : [ShutdownError == true]
  Error -> OFF [order 2] : [ShutdownError == false &&...
      | KL15==false]
  OFF -> Error [order 2] : [ShutdownError == true]
  data: CMState output uint8; KL15 input; FL_boREQ_MainHV_ON_MINUS input; KL15_AllBoxes input; BattRelay_Closed input; MainHV_Plus_Status input; InsulationReadyOK input; BattRelay_Close_Req input; REQ_IMD_ON input; ShutdownError input; IMD_Available input

== stateflow chart ChiefMaster_TTC580/ChiefMaster/Flow Logic/System Status/EmergencySD/Emergency_Switch_Control/EmergencySwitch_Input_Delay ==
  state Initial
    out = IP_boVS_EmergensySwitch;
  state Delay
    out = true;
  state After_delay
    out = IP_boVS_EmergensySwitch;
  (default) -> Initial
  After_delay -> Initial : [IP_boVS_EmergensySwitch == true]
  Initial -> Delay : [IP_boVS_EmergensySwitch == false]
  Delay -> After_delay : [after(10, msec)]
  data: IP_boVS_EmergensySwitch input; out output

== stateflow chart ChiefMaster_TTC580/ChiefMaster/Input Processing/HW Inputs/Subsystem1/Input_Delay ==
  state Initial
    out = true;
  state After_delay
    out = Input;
  (default) -> Initial
  Initial -> After_delay : [after(IP_u8HW_IN_delay_ms, msec)]
  data: out output; IP_u8HW_IN_delay_ms input; Input input

== stateflow chart ChiefMaster_TTC580/ChiefMaster/Input Processing/HW Inputs/Subsystem2/Input_Delay ==
  state Initial
    out = true;
  state After_delay
    out = Input;
  (default) -> Initial
  Initial -> After_delay : [after(IP_u8HW_IN_delay_ms, msec)]
  data: out output; IP_u8HW_IN_delay_ms input; Input input

== stateflow chart ChiefMaster_TTC580/ChiefMaster/Flow Logic/System Status/SDError/Chart ==
  state Default
    System_Error = false;
  state Error
    System_Error = true;
  (default) -> Default
  Error -> Default : [KL15_CM_reset == true]
  Default -> Error : [In == true]
  data: In input; System_Error output; KL15_CM_reset input

== stateflow chart ChiefMaster_TTC580/ChiefMaster/Flow Logic/System Status/SDError/Subsystem/Chart ==
  state Default
    Out = false
  state hold
    Out = false
  state Actual
    Out = REQ_HV_ON_BB
  (default) -> Default
  Default -> hold : [In == true]
  Actual -> Default : [KL15_CM_Reset == true]
  hold -> Actual : [after(5,sec)]
  data: In input; Out output; REQ_HV_ON_BB input; KL15_CM_Reset input

== stateflow chart ChiefMaster_TTC580/ChiefMaster/Flow Logic/System Status/SDError/Subsystem/Chart1 ==
  state Default
    Out = false
  state hold
    Out = false
  state Actual
    Out = REQ_HV_ON_BB
  (default) -> Default
  Default -> hold : [In == true]
  Actual -> Default : [KL15_CM_Reset == true]
  hold -> Actual : [after(5,sec)]
  data: In input; Out output; REQ_HV_ON_BB input; KL15_CM_Reset input

== stateflow chart ChiefMaster_TTC580/ChiefMaster/Flow Logic/System Status/SDError/Subsystem/Chart2 ==
  state Default
    Out = false
  state hold
    Out = false
  state Actual
    Out = REQ_HV_ON_BB
  (default) -> Default
  Default -> hold : [In == true]
  Actual -> Default : [KL15_CM_Reset == true]
  hold -> Actual : [after(5,sec)]
  data: In input; Out output; REQ_HV_ON_BB input; KL15_CM_Reset input

== stateflow chart ChiefMaster_TTC580/ChiefMaster/Flow Logic/BDU Control/BDUSystem/Subsystem1/Chart4 ==
  state Default
    Out = false
  state Default1
    Out = true
  (default) -> Default
  Default1 -> Default : [WeldingDetection_Status == 1 ||...
      | WeldingDetection_Status == 2]
  Default -> Default1 : [In == true]
  data: In input boolean; Out output boolean; WeldingDetection_Status input uint8

== stateflow chart ChiefMaster_TTC580/ChiefMaster/Flow Logic/BDU Control/BDUSystem/Subsystem2/Chart_WeldingDetection ==
  state Default
    REQ_MainHV_ON_PLUS = false
    REQ_MainHV_ON_MINUS = false
    MainHV_Minus_Welded = false
    MainHV_Plus_Welded = false
    WeldingDetection_Status = uint8(0);
  state Open
    REQ_MainHV_ON_PLUS = false
    REQ_MainHV_ON_MINUS = false
    MainHV_Minus_Welded = false
    MainHV_Plus_Welded = false
  state Error
    MainHV_Minus_Welded = true
    MainHV_Plus_Welded = true
    WeldingDetection_Status = uint8(2);
  state Plus_Close
    REQ_MainHV_ON_PLUS = true
  state ErrorMinus
    MainHV_Minus_Welded = true
    WeldingDetection_Status = uint8(2);
  state Minus_Close
    REQ_MainHV_ON_MINUS = true
  state ErrorVoltage
    WeldingDetection_Status = uint8(2);
  state Default3
    REQ_MainHV_ON_PLUS = false
  state ErrorPlus
    MainHV_Plus_Welded = true
    WeldingDetection_Status = uint8(2);
  state Open1
    REQ_MainHV_ON_PLUS = false
    REQ_MainHV_ON_MINUS = false
    MainHV_Minus_Welded = false
    MainHV_Plus_Welded = false
    WeldingDetection_Status = uint8(1);
  (default) -> Default
  Default -> Open : [In == true]
  Open1 -> Open : [In == true]
  Open -> Error [order 2] : after(5,sec)
  Open -> Plus_Close [order 1] : [LoadVtg <= 20]
  Plus_Close -> ErrorMinus [order 2] : after(5,sec)
  Plus_Close -> Minus_Close [order 1] : [LoadVtg <= 20]
  Minus_Close -> ErrorVoltage [order 2] : after(5,sec)
  Minus_Close -> Default3 [order 1] : [abs(LoadVtg - SystemVtg) <= 5]
  Default3 -> ErrorPlus [order 1] : after(5,sec)
  Default3 -> Open1 [order 2] : [LoadVtg <= 20]
  data: LoadVtg input single; SystemVtg input single; MainHV_Minus_Welded output boolean; MainHV_Plus_Welded output boolean; REQ_MainHV_ON_MINUS output boolean; REQ_MainHV_ON_PLUS output boolean; In input boolean; WeldingDetection_Status output uint8

== stateflow chart ChiefMaster_TTC580/ChiefMaster/Flow Logic/System Status/AlarmBuzzer/Chart ==
  state BuzzerON
    out=true;
  state BuzzerOFF
    out=false;
  (default) -> BuzzerON
  BuzzerON -> BuzzerOFF : [after(BuzzerTimer,sec)]
  data: BuzzerTimer input; out output

== stateflow chart ChiefMaster_TTC580/ChiefMaster/Flow Logic/System Status/EMSRET_Power/EMSRET ==
  state OFF
    EMSRET=false;
  state ON
    EMSRET=true;
  state ShutOff
    EMSRET=false;
  state Delay
    EMSRET=true;
  (default) -> OFF
  OFF -> ON : [AllOK==true]
  ShutOff -> OFF : [Reset==true]
  ON -> Delay : [AllOK==false]
  Delay -> ShutOff : [after(3,sec)]
  data: AllOK input; Reset input; EMSRET output

== stateflow chart ChiefMaster_TTC580/ChiefMaster/Flow Logic/BDU Control/BDUSystem/delay1 ==
  state Default
    Out = false
  state hold
    Out = false
  state Actual
    Out = In
  (default) -> Default
  (junction 15) -> Default : [In == false]
  Default -> hold : [In == true]
  hold -> (junction 15) [order 2]
  Actual -> (junction 15)
  hold -> Actual [order 1] : after(DelayTime_ms,msec)
  data: In input boolean; Out output boolean; DelayTime_ms input
